simulink model "symulacja2012_serv"  (Simulink 7.9)
settings: Solver=ode4  SolverMode=SingleTasking  StartTime=0.0  StopTime=5000.0  FixedStep=0.1  RelTol=1e-3
values from neighbouring files (symbols this model uses):
  cb = 1000    [run.m]    (also in run_rs.m; run_serv.m; run_sim.m; with_server.m)
  ch = 2700    [run.m]    (also in run_rs.m; run_serv.m; run_sim.m; with_server.m)
  cw = 4200    [run.m]    (also in run_rs.m; run_serv.m; run_sim.m; with_server.m)
  cwym = 2700    [run.m]    (also in run_rs.m; run_serv.m; run_sim.m; with_server.m)
  dz = 1000    [run.m]    (also in run_rs.m; run_serv.m; run_sim.m; with_server.m)
  kext = 15000    [run.m]    (also in run_rs.m; run_serv.m; run_sim.m; with_server.m)
  kh = 12000    [run.m]    (also in run_rs.m; run_serv.m; run_sim.m; with_server.m)
  kw = 250000    [run.m]    (also in run_rs.m; run_serv.m; run_sim.m; with_server.m)
  mb = 20000    [run.m]    (also in run_rs.m; run_serv.m; run_sim.m; with_server.m)
  mco = 3000    [run.m]    (also in run_rs.m; run_serv.m; run_sim.m; with_server.m)
  mh = 3000    [run.m]    (also in run_rs.m; run_serv.m; run_sim.m; with_server.m)
  mm = 3000    [run.m]    (also in run_rs.m; run_serv.m; run_sim.m; with_server.m)
  To = 5    [run.m]    (also in run_rs.m; run_serv.m; run_sim.m = -30; with_server.m = ???)
  Tpco1_in = 5    [run.m]    (also in run_rs.m; run_sim.m)
  Tpco2_in = 5    [run.m]    (also in run_rs.m; run_sim.m)
  Tpm_in = 5    [run.m]    (also in run_rs.m; run_sim.m)
  Tr1_in = 5    [run.m]    (also in run_rs.m; run_sim.m)
  Tr2_in = 5    [run.m]    (also in run_rs.m; run_sim.m)
  Tzco_in = 5    [run.m]    (also in run_rs.m; run_sim.m)
undefined symbols (not defined in the file or in its folder): Ub1, Ub2, Um
settings Model: Creator=Piotr  LastModifiedBy=student
settings OptimizationCC: BlockReduction=off  BooleanDataType=off
settings DebuggingCC: SaveWithParameterizedLinksMsg=none  SignalResolutionControl=TryResolveAllWithWarning  SolverPrmCheckMsg=none  MultiTaskDSMMsg=warning  MultiTaskCondExecSysMsg=none  FrameProcessingCompatibilityMsg=error
settings HardwareCC: TargetUnknown=on
settings CodeAppCC: CustomSymbolStrType=$N$R$M_T
settings GRTTargetCC: CodeReplacementLibrary=C89/C90 (ANSI)

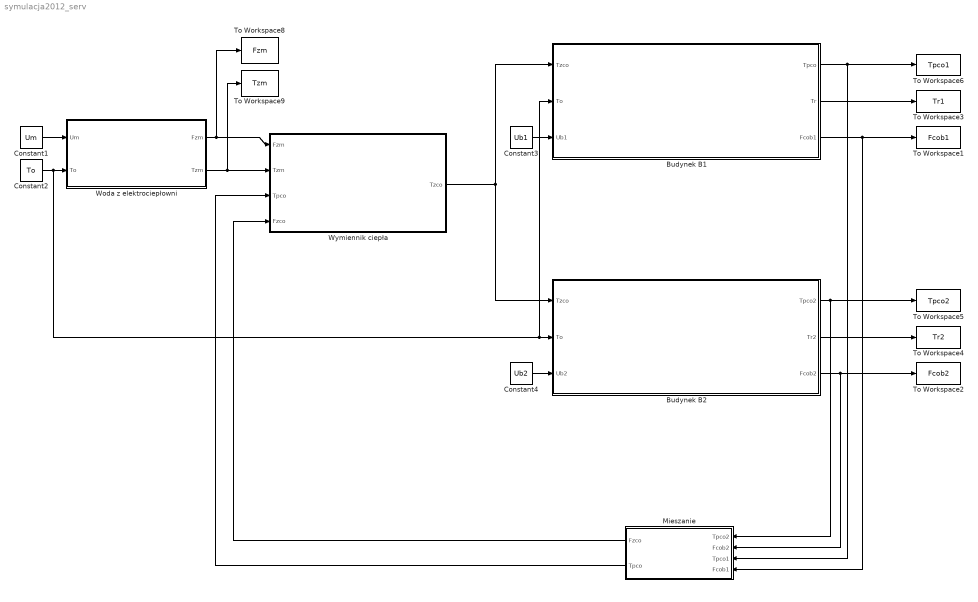
== system symulacja2012_serv ==
  Budynek B1 : Subsystem
  Budynek B2 : Subsystem
  Constant1 : Constant  Value=Um
  Constant2 : Constant  Value=To
  Constant3 : Constant  Value=Ub1
  Constant4 : Constant  Value=Ub2
  Mieszanie : Subsystem
  To Workspace1 : ToWorkspace  VariableName=Fcob1  SampleTime=-1
  To Workspace2 : ToWorkspace  VariableName=Fcob2  SampleTime=-1
  To Workspace3 : ToWorkspace  VariableName=Tr1  SampleTime=-1
  To Workspace4 : ToWorkspace  VariableName=Tr2  SampleTime=-1
  To Workspace5 : ToWorkspace  VariableName=Tpco2  SampleTime=-1
  To Workspace6 : ToWorkspace  VariableName=Tpco1  SampleTime=-1
  To Workspace8 : ToWorkspace  VariableName=Fzm  SampleTime=-1
  To Workspace9 : ToWorkspace  VariableName=Tzm  SampleTime=-1
  Woda z elektrociepłowni : Subsystem
  Wymiennik ciepła : Subsystem
  wires:
  Budynek B2/1(Tpco2) -> Mieszanie/1(Tpco2), To Workspace5/1
  Budynek B2/2(Tr2) -> To Workspace4/1
  Budynek B1/2(Tr) -> To Workspace3/1
  Budynek B1/1(Tpco) -> Mieszanie/3(Tpco1), To Workspace6/1
  Woda z elektrociepłowni/1(Fzm) -> To Workspace8/1, Wymiennik ciepła/1(Fzm)
  Woda z elektrociepłowni/2(Tzm) -> Wymiennik ciepła/2(Tzm), To Workspace9/1
  Constant2/1 -> Budynek B2/2(To), Budynek B1/2(To), Woda z elektrociepłowni/2(To)
  Budynek B2/3("Fcob2 ") -> To Workspace2/1, Mieszanie/2(Fcob2)
  Mieszanie/2(Tpco) -> Wymiennik ciepła/3(Tpco)
  Mieszanie/1(Fzco) -> Wymiennik ciepła/4(Fzco)
  Budynek B1/3("Fcob1 ") -> Mieszanie/4("Fcob1 "), To Workspace1/1
  Wymiennik ciepła/1(Tzco) -> Budynek B1/1(Tzco), Budynek B2/1(Tzco)
  Constant1/1 -> Woda z elektrociepłowni/1(Um)
  Constant4/1 -> Budynek B2/3(Ub2)
  Constant3/1 -> Budynek B1/3(Ub1)

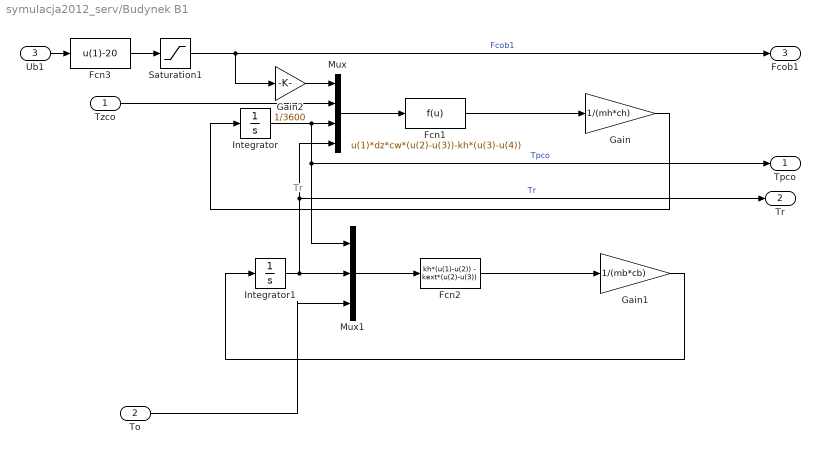
== system symulacja2012_serv/Budynek B1 ==
  note: Tr
  Tzco : Inport
  To : Inport  Port=2
  Ub1 : Inport  Port=3
  Fcn1 : Fcn  Expr=u(1)*dz*cw*(u(2)-u(3))-kh*(u(3)-u(4))
  Fcn2 : Fcn  Expr=kh*(u(1)-u(2)) - kext*(u(2)-u(3))
  Fcn3 : Fcn  Expr=u(1)-20
  Gain : Gain  Gain=1/(mh*ch)
  Gain1 : Gain  Gain=1/(mb*cb)
  Gain2 : Gain  Gain=1/3600
  Integrator : Integrator  InitialCondition=Tpco1_in
  Integrator1 : Integrator  InitialCondition=Tr1_in
  Mux : Mux
  Mux1 : Mux  Inputs=3
  Saturation1 : Saturate  UpperLimit=40  LowerLimit=0
  Tpco : Outport
  Tr : Outport  Port=2
  "Fcob1 " : Outport  Port=3
  wires:
  Integrator/1 -> Mux1/1, Tpco/1, Mux/3  "Tpco"
  Integrator1/1 -> Mux1/2, Tr/1, Mux/4  "Tr"
  Gain1/1 -> Integrator1/1
  Fcn2/1 -> Gain1/1
  Mux1/1 -> Fcn2/1
  To/1 -> Mux1/3
  Gain/1 -> Integrator/1
  Fcn1/1 -> Gain/1
  Mux/1 -> Fcn1/1
  Tzco/1 -> Mux/2
  Fcn3/1 -> Saturation1/1
  Ub1/1 -> Fcn3/1
  Saturation1/1 -> "Fcob1 "/1, Gain2/1  "Fcob1"
  Gain2/1 -> Mux/1

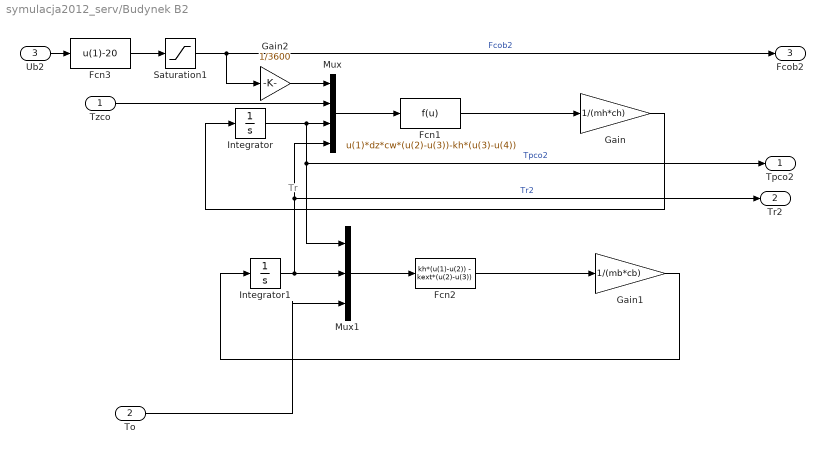
== system symulacja2012_serv/Budynek B2 ==
  note: Tr
  Tzco : Inport
  To : Inport  Port=2
  Ub2 : Inport  Port=3
  Fcn1 : Fcn  Expr=u(1)*dz*cw*(u(2)-u(3))-kh*(u(3)-u(4))
  Fcn2 : Fcn  Expr=kh*(u(1)-u(2)) - kext*(u(2)-u(3))
  Fcn3 : Fcn  Expr=u(1)-20
  Gain : Gain  Gain=1/(mh*ch)
  Gain1 : Gain  Gain=1/(mb*cb)
  Gain2 : Gain  Gain=1/3600
  Integrator : Integrator  InitialCondition=Tpco2_in
  Integrator1 : Integrator  InitialCondition=Tr2_in
  Mux : Mux
  Mux1 : Mux  Inputs=3
  Saturation1 : Saturate  UpperLimit=40  LowerLimit=0
  Tpco2 : Outport
  Tr2 : Outport  Port=2
  "Fcob2 " : Outport  Port=3
  wires:
  Integrator/1 -> Mux1/1, Tpco2/1, Mux/3  "Tpco2"
  Integrator1/1 -> Mux1/2, Tr2/1, Mux/4  "Tr2"
  Gain1/1 -> Integrator1/1
  Fcn2/1 -> Gain1/1
  Mux1/1 -> Fcn2/1
  To/1 -> Mux1/3
  Gain/1 -> Integrator/1
  Fcn1/1 -> Gain/1
  Mux/1 -> Fcn1/1
  Tzco/1 -> Mux/2
  Fcn3/1 -> Saturation1/1
  Ub2/1 -> Fcn3/1
  Saturation1/1 -> "Fcob2 "/1, Gain2/1  "Fcob2"
  Gain2/1 -> Mux/1

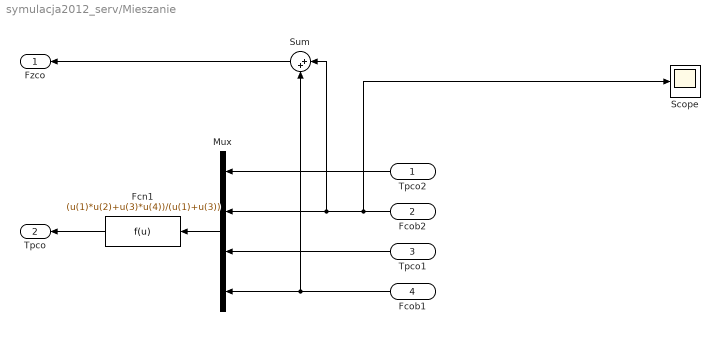
== system symulacja2012_serv/Mieszanie ==
  Tpco2 : Inport
  Fcob2 : Inport  Port=2
  Tpco1 : Inport  Port=3
  "Fcob1 " : Inport  Port=4
  Fcn1 : Fcn  Expr=(u(1)*u(2)+u(3)*u(4))/(u(1)+u(3))
  Mux : Mux
  Scope : Scope
      settings: YMin=-1.00000  YMax=1.00000
  Sum : Sum  Inputs=|++
  Fzco : Outport
  Tpco : Outport  Port=2
  wires:
  Mux/1 -> Fcn1/1
  Fcn1/1 -> Tpco/1
  Tpco2/1 -> Mux/1
  Tpco1/1 -> Mux/3
  "Fcob1 "/1 -> Sum/2, Mux/4
  Fcob2/1 -> Scope/1, Sum/1, Mux/2
  Sum/1 -> Fzco/1

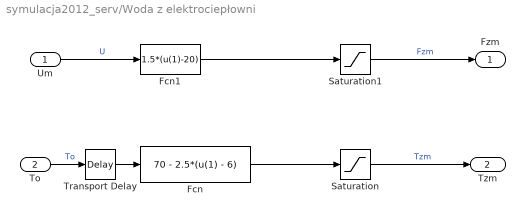
== system symulacja2012_serv/Woda z elektrociepłowni ==
  Um : Inport
  To : Inport  Port=2
  Fcn : Fcn  Expr=70 - 2.5*(u(1) - 6)
  Fcn1 : Fcn  Expr=1.5*(u(1)-20)
  Saturation : Saturate  UpperLimit=135  LowerLimit=70
  Saturation1 : Saturate  UpperLimit=80  LowerLimit=0
  Transport Delay : TransportDelay  DelayTime=8
  Fzm : Outport
  Tzm : Outport  Port=2
  wires:
  Um/1 -> Fcn1/1  "U"
  Saturation/1 -> Tzm/1  "Tzm"
  Saturation1/1 -> Fzm/1  "Fzm"
  To/1 -> Transport Delay/1  "To"
  Fcn/1 -> Saturation/1
  Fcn1/1 -> Saturation1/1
  Transport Delay/1 -> Fcn/1

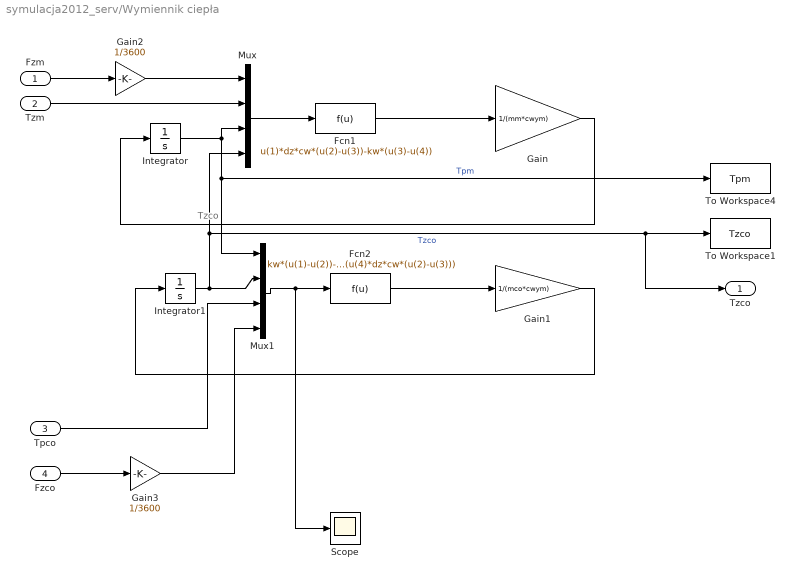
== system symulacja2012_serv/Wymiennik ciepła ==
  note: Tzco
  Fzm : Inport
  Tzm : Inport  Port=2
  Tpco : Inport  Port=3
  Fzco : Inport  Port=4
  Fcn1 : Fcn  Expr=u(1)*dz*cw*(u(2)-u(3))-kw*(u(3)-u(4))
  Fcn2 : Fcn  Expr=kw*(u(1)-u(2))-(u(4)*dz*cw*(u(2)-u(3)))
  Gain : Gain  Gain=1/(mm*cwym)
  Gain1 : Gain  Gain=1/(mco*cwym)
  Gain2 : Gain  Gain=1/3600
  Gain3 : Gain  Gain=1/3600
  Integrator : Integrator  InitialCondition=Tpm_in
  Integrator1 : Integrator  InitialCondition=Tzco_in
  Mux : Mux
  Mux1 : Mux
  Scope : Scope
      settings: SaveName=ScopeData3  MaxDataPoints=50000
  To Workspace1 : ToWorkspace  VariableName=Tzco  SampleTime=-1
  To Workspace4 : ToWorkspace  VariableName=Tpm  SampleTime=-1
  Tzco : Outport
  wires:
  Gain/1 -> Integrator/1
  Mux1/1 -> Fcn2/1, Scope/1
  Gain1/1 -> Integrator1/1
  Tpco/1 -> Mux1/3
  Integrator1/1 -> Mux1/2, Mux/4, Tzco/1, To Workspace1/1  "Tzco"
  Integrator/1 -> To Workspace4/1, Mux1/1, Mux/3  "Tpm"
  Tzm/1 -> Mux/2
  Mux/1 -> Fcn1/1
  Fcn1/1 -> Gain/1
  Fcn2/1 -> Gain1/1
  Fzm/1 -> Gain2/1
  Fzco/1 -> Gain3/1
  Gain2/1 -> Mux/1
  Gain3/1 -> Mux1/4
